simulink model "Z3"  (R2017b)
settings: Solver=VariableStepAuto  StartTime=0.0  StopTime=50.0  RelTol=1e-3
settings Model: Creator=Mahe  LastModifiedBy=Mahe

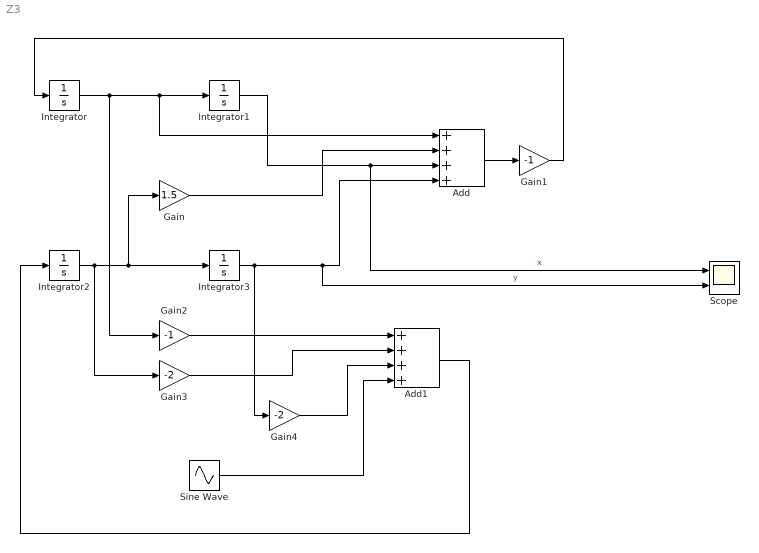
== system Z3 ==
  Add : Sum  Inputs=4
  Add1 : Sum  Inputs=4
  Gain : Gain  Gain=1.5
  Gain1 : Gain  Gain=-1
  Gain2 : Gain  Gain=-1
  Gain3 : Gain  Gain=-2
  Gain4 : Gain  Gain=-2
  Integrator : Integrator
  Integrator1 : Integrator
  Integrator2 : Integrator  InitialCondition=-1
  Integrator3 : Integrator  InitialCondition=1
  Scope : Scope  NumInputPorts=2
  Sine Wave : Sin  Frequency=3.14  SampleTime=0
  wires:
  Integrator/1 -> Gain2/1, Add/1, Integrator1/1
  Integrator2/1 -> Gain3/1, Gain/1, Integrator3/1
  Integrator3/1 -> Gain4/1, Scope/2, Add/4  "y"
  Integrator1/1 -> Scope/1, Add/3  "x"
  Gain/1 -> Add/2
  Add/1 -> Gain1/1
  Gain1/1 -> Integrator/1
  Gain2/1 -> Add1/1
  Gain3/1 -> Add1/2
  Gain4/1 -> Add1/3
  Sine Wave/1 -> Add1/4
  Add1/1 -> Integrator2/1
